simulink model "proj"  (R2022b)
settings: Solver=VariableStepAuto  StartTime=0.0  StopTime=0.01  RelTol=1e-3
undefined symbols (not defined in the file): Ion, Lithium
libraries: spsSeriesRLCBranchLib x3, spsBatteryLib x2, spsMosfetLib x2, spsCurrentMeasurementLib x1, spsVoltageMeasurementLib x1, spspowerguiLib x1
settings Model: Creator=gobis  LastModifiedBy=gobis
settings SolverCC: ZeroCrossAlgorithm=Adaptive
settings DebuggingCC: IgnoredZcDiagnostic=none

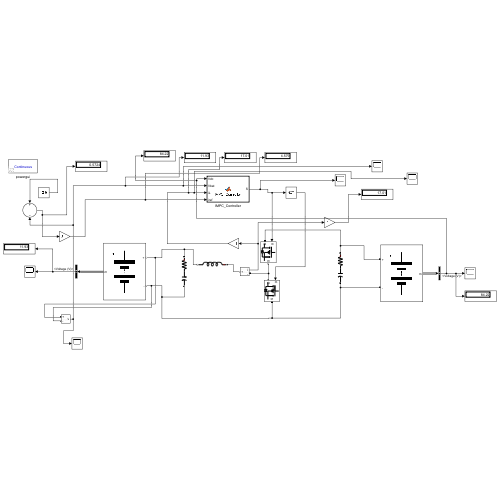
[thumbnail: Simulink's stored preview of the top-level diagram]
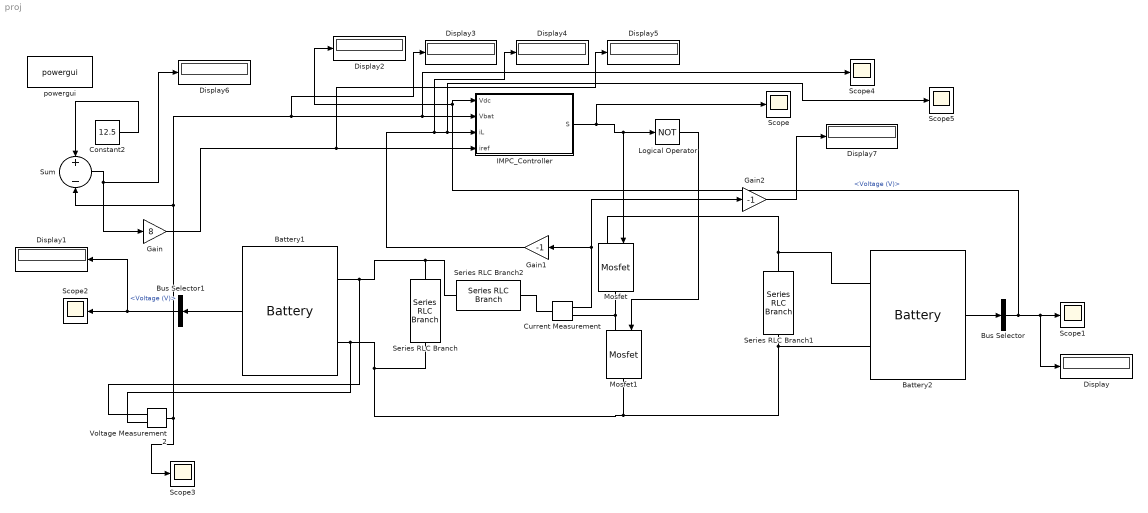
== system proj ==
  Battery1 : spsBatteryLib/Battery  BatType=Lithium-Ion  ShowTempParam=off  ThermalPreset=no  ShowAgeParam=off  NomV=10  NomQ=7  SOC=100  Batt_Tr=30  PresetModel=on  MaxQ=7  MinV=7.5  FullV=11.6399  Dis_rate=3.0435  R=0.014286  Normal_OP=6.3304  expZone="[10.8039     0.343913]"  current=[6.5 13 32.5]  Units=Time  Tci=20  NomT=20  T2=-30  MaxQ2=4.8  FullV2=7.1  Normal_OP2=5.655  expZone2="[6.58           1]"  Rca=0.6  ti=2000  Dp=0  Neq0=0  Tsim=1e6  Ta1=25  Qeol=5.4*0.9  Reol=0.013333*1.2  Char_age=[2.3478, 3]  Dis_age=[2.3478, 10]  N1=1500  N2=10500  N3=1000  N4=1400  Ta2=45  N5=950
  Battery2 : spsBatteryLib/Battery  BatType=Lithium-Ion  ShowTempParam=off  ThermalPreset=no  ShowAgeParam=off  NomV=80  NomQ=7  SOC=50  Batt_Tr=30  PresetModel=on  MaxQ=7  MinV=60  FullV=93.119  Dis_rate=3.0435  R=0.11429  Normal_OP=6.3304  expZone="[86.4309     0.343913]"  current=[6.5 13 32.5]  Units=Time  Tci=20  NomT=20  T2=-30  MaxQ2=4.8  FullV2=7.1  Normal_OP2=5.655  expZone2="[6.58           1]"  Rca=0.6  ti=2000  Dp=0  Neq0=0  Tsim=1e6  Ta1=25  Qeol=5.4*0.9  Reol=0.013333*1.2  Char_age=[2.3478, 3]  Dis_age=[2.3478, 10]  N1=1500  N2=10500  N3=1000  N4=1400  Ta2=45  N5=950
  Bus Selector : BusSelector  OutputSignals=Voltage (V)
  Bus Selector1 : BusSelector  OutputSignals=Voltage (V)
  Constant2 : Constant  Value=12.5
  Current Measurement : spsCurrentMeasurementLib/Current Measurement  PhasorSimulation=off  OutputType=Complex  PSBequivalent=0
  Display{,1..7} (8 alike) : Display
  Gain : Gain  Gain=8
  Gain1 : Gain  Gain=-1
  Gain2 : Gain  Gain=-1
  IMPC_Controller : MATLAB Function  TreatAsAtomicUnit=on
  Logical Operator : Logic  Operator=NOT  AllPortsSameDT=off  OutDataTypeStr=boolean
  Mosfet : spsMosfetLib/Mosfet  Ron=0.1  Lon=0  Rd=0.01  Vfd=0  IC=0  Rs=1e5  Cs=inf  Measurements=off
  Mosfet1 : spsMosfetLib/Mosfet  Ron=0.1  Lon=0  Rd=0.01  Vfd=0  IC=0  Rs=1e5  Cs=inf  Measurements=off
  Scope{,1..5} (6 alike) : Scope
  Series RLC Branch : spsSeriesRLCBranchLib/Series RLC Branch  LConnTagsString=__new0  RConnTagsString=__new0  BranchType=RC  Resistance=1  Inductance=1e-3  SetiL0=off  InitialCurrent=0  Capacitance=1e-6  Setx0=off  InitialVoltage=0  Measurements=None
  Series RLC Branch1 : spsSeriesRLCBranchLib/Series RLC Branch  LConnTagsString=__new0  RConnTagsString=__new0  BranchType=RC  Resistance=1  Inductance=1e-3  SetiL0=off  InitialCurrent=0  Capacitance=1e-6  Setx0=off  InitialVoltage=0  Measurements=None
  Series RLC Branch2 : spsSeriesRLCBranchLib/Series RLC Branch  LConnTagsString=__new0  RConnTagsString=__new0  BranchType=L  Resistance=1  Inductance=1e-3  SetiL0=off  InitialCurrent=0  Capacitance=1e-6  Setx0=off  InitialVoltage=0  Measurements=None
  Sum : Sum  Inputs=+-
  Voltage Measurement2 : spsVoltageMeasurementLib/Voltage Measurement  PhasorSimulation=off  OutputType=Complex  PSBequivalent=0
  powergui : spspowerguiLib/powergui  Priority=1  SimulationMode=Continuous  SampleTime=50e-6  frequency=60  Iterations=50  frequencyindice=0  Pbase=100e6  ErrMax=1e-4  UnitsV=kV  UnitsW=MW  buscounter=0  FunctionMessages=off  echomessages=off  EnableUseOfTLC=off  CurrentSourceSwitches=off  DisableSnubberDevices=off  DisableRonSwitches=off  DisableVfSwitches=off  DisplayEquations=off  AutomaticDiscreteSolvers=off  SolverType=Tustin/Backward Euler (TBE)  Interpol=off  ExternalGateDelay=off  methode=off  Ts=100  x0status=blocks  SPID=on  SwTol=0  HookPort=off  NonlinearTolerance=1e-4  nMaxIteration=100  ContinueOnMaxIteration=off  RestoreLinks=warning  ResistiveCurrentMeasurement=off  Frange=[0:2:500]  Ylog=off  Xlog=on  ShowGrid=off  save=off  variable=ZData  structure=0  ZoomFFT=off  StartTime=0.0  cycles=1  DisplayStyle=1  fundamental=60  FreqAxis=off  MaxFrequency=1000  frequencyindicesteady=1  RmsSteady=1  display=off
  wires:
  Battery2/1 -> Bus Selector/1
  Bus Selector/1 -> Display2/1, IMPC_Controller/1(Vdc), Display/1, Scope1/1  "<Voltage (V)>"
  Bus Selector1/1 -> Scope2/1, Display1/1  "<Voltage (V)>"
  Battery1/1 -> Bus Selector1/1
  Current Measurement/1 -> Gain2/1, Gain1/1
  Constant2/1 -> Sum/1
  Sum/1 -> Gain/1, Display6/1
  Gain/1 -> Display5/1, IMPC_Controller/4(iref)
  IMPC_Controller/1(S) -> Scope/1, Mosfet/1, Logical Operator/1
  Logical Operator/1 -> Mosfet1/1
  Voltage Measurement2/1 -> Display3/1, Scope4/1, IMPC_Controller/2(Vbat), Sum/2, Scope3/1
  Gain1/1 -> Display4/1, Scope5/1, IMPC_Controller/3(iL)
  Gain2/1 -> Display7/1
  connections:
  Series RLC Branch/LConn1 -- Voltage Measurement2/LConn1 -- Battery1/LConn1 -- Series RLC Branch2/RConn1
  Series RLC Branch1/LConn1 -- Battery2/LConn1 -- Mosfet/LConn1
  Battery1/LConn2 -- Voltage Measurement2/LConn2 -- Battery2/LConn2 -- Series RLC Branch1/RConn1 -- Mosfet1/RConn1 -- Series RLC Branch/RConn1
  Mosfet1/LConn1 -- Mosfet/RConn1 -- Current Measurement/RConn1
  Current Measurement/LConn1 -- Series RLC Branch2/LConn1

== matlab function proj/IMPC_Controller ==
  settings: updateMethod=DISCRETE
  data: Vdc input; S output; Vbat input; iL input; iref input
function S = IMPC_Controller(Vdc,Vbat,iL,iref)

Ts = 1e-5;
L  = 1e-3;

Imax = 10;

persistent u_prev

if isempty(u_prev)
    u_prev = 0;
end

Jmin = inf;
S = 0;

for u = 0:1

    if u == 1
        i_pred = iL + (Ts/L)*(Vdc - Vbat);
    else
        i_pred = iL - (Ts/L)*Vbat;
    end

    if abs(i_pred) > Imax

        J = 1e12;

    else

        w1 = 1;
        w2 = 0.5;
        w3 = 0.01;

        J = w1*(iref - i_pred)^2 ...
          + w2*(i_pred - iL)^2 ...
          + w3*(u - u_prev)^2;

    end

    if J < Jmin
        Jmin = J;
        S = u;
    end

end

u_prev = S;

end
